simulink model "scd3busMicrogridDroopControlFidelityLevels3Inv"  (R2025b)
settings: Solver=ode15s  StartTime=0.0  StopTime=24  RelTol=1e-3
PreLoadFcn:
  | scd3busMicrogridDroopControlDataFidelityLevels3Inv;
  | 
  | %% Controller variants
  | % Create variant controls for converter controller. Controller has two
  | % different levels of fidelity: Averaged, AveragedPulse, Pulse
  | Averaged = Simulink.VariantExpression;
  | Averaged.Condition = 'fidelity==scd3busMicrogridDroopControl_variants_enum.Low';
  | Pulse = Simulink.VariantExpression;
  | Pulse.Condition = 'fidelity==scd3busMicrogridDroopControl_variants_enum.High';
  | 
  | %% Plant variants
  | % Create variant controls for converter plant. Plant has three different
  | % levels of fidelity.
  | AveragedNonSwitch = Simulink.VariantExpression;
  | AveragedNonSwitch.Condition = 'fidelity==scd3busMicrogridDroopControl_variants_enum.Low';
  | PulseSwitch = Simulink.VariantExpression;
  | PulseSwitch.Condition = 'fidelity==scd3busMicrogridDroopControl_variants_enum.High';
  | 
  | %% Set up variables ready for simulation
  | fidelity = scd3busMicrogridDroopControl_variants_enum.High;
  | Ts = 5e-6;
  | Ts_V = 1e-6;
  | Tsc = 1e-4;
  | Tsc_V = 5e-4;
values from neighbouring files (symbols this model uses):
  consensus_enable = 1    [scd3busMicrogridDroopControlDataFidelityLevels3Inv.m]
  fgrid = 60    [scd3busMicrogridDroopControlDataFidelityLevels.m]    (also in scd3busMicrogridDroopControlDataFidelityLevels3Inv.m)
  Kdroop_fp1 = 0.03/2    (= 0.015)    [scd3busMicrogridDroopControlDataFidelityLevels3Inv.m]
  Kdroop_fp2 = 0.03/2    (= 0.015)    [scd3busMicrogridDroopControlDataFidelityLevels3Inv.m]
  Kdroop_vq1 = 0.05/2    (= 0.025)    [scd3busMicrogridDroopControlDataFidelityLevels3Inv.m]
  Kdroop_vq2 = 0.05/2    (= 0.025)    [scd3busMicrogridDroopControlDataFidelityLevels3Inv.m]
  Ki_vd = 850    [scd3busMicrogridDroopControlDataFidelityLevels.m]    (also in scd3busMicrogridDroopControlDataFidelityLevels3Inv.m)
  Ki_vq = 850    [scd3busMicrogridDroopControlDataFidelityLevels.m]    (also in scd3busMicrogridDroopControlDataFidelityLevels3Inv.m)
  Kp_vd = 0.36    [scd3busMicrogridDroopControlDataFidelityLevels.m]    (also in scd3busMicrogridDroopControlDataFidelityLevels3Inv.m)
  Kp_vq = 0.36    [scd3busMicrogridDroopControlDataFidelityLevels.m]    (also in scd3busMicrogridDroopControlDataFidelityLevels3Inv.m)
  Vdc1 = 1000    [scd3busMicrogridDroopControlDataFidelityLevels.m]    (also in scd3busMicrogridDroopControlDataFidelityLevels3Inv.m)
  Vdc2 = 1000    [scd3busMicrogridDroopControlDataFidelityLevels.m]    (also in scd3busMicrogridDroopControlDataFidelityLevels3Inv.m)
  Vrms = 380    [scd3busMicrogridDroopControlDataFidelityLevels.m]    (also in scd3busMicrogridDroopControlDataFidelityLevels3Inv.m)
undefined symbols (not defined in the file or in its folder): DiscIntNeverNeededParam
libraries: ee_lib x29, nesl_utility x27, fl_lib x15, eeTransforms x4, eeSinusoidalMeasurement x4, slpidlib x4, eePwmGeneratorTwoLevel x2, eePowerMeasurement x2, simulink x2, SignalEditorBlockLib x1
(part 1 of 3)
Description:
  | Three-Phase 3 Bus Low-Inertia Microgrid Droop Control Example
settings Model: SimulationMode=rapid-accelerator  Creator=The MathWorks, Inc.  LastModifiedBy=Alex
settings SolverCC: MaxZcPerStep=1.0
settings DataIOCC: SaveOutput=off  DSMLogging=off  SaveTime=off  ReturnWorkspaceOutputs=off
settings OptimizationCC: ReuseModelBlockBuffer=off
settings DebuggingCC: StateNameClashWarn=warning
settings ModelReferenceCC: EnableRefExpFcnMdlSchedulingChecks=on
settings RTWCC: GPUComputeCapability=3.5
settings SimscapeCC: SimscapeNormalizeSystem=off

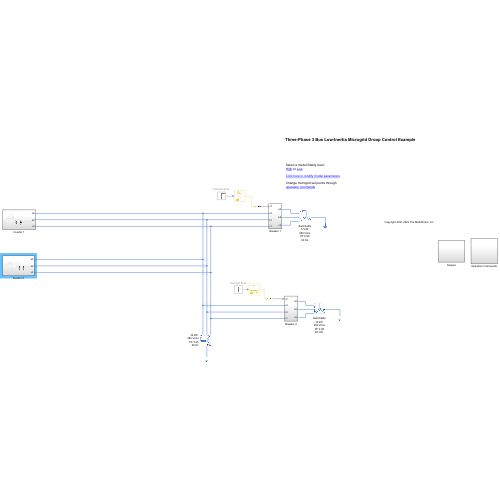
[thumbnail: Simulink's stored preview of the top-level diagram]
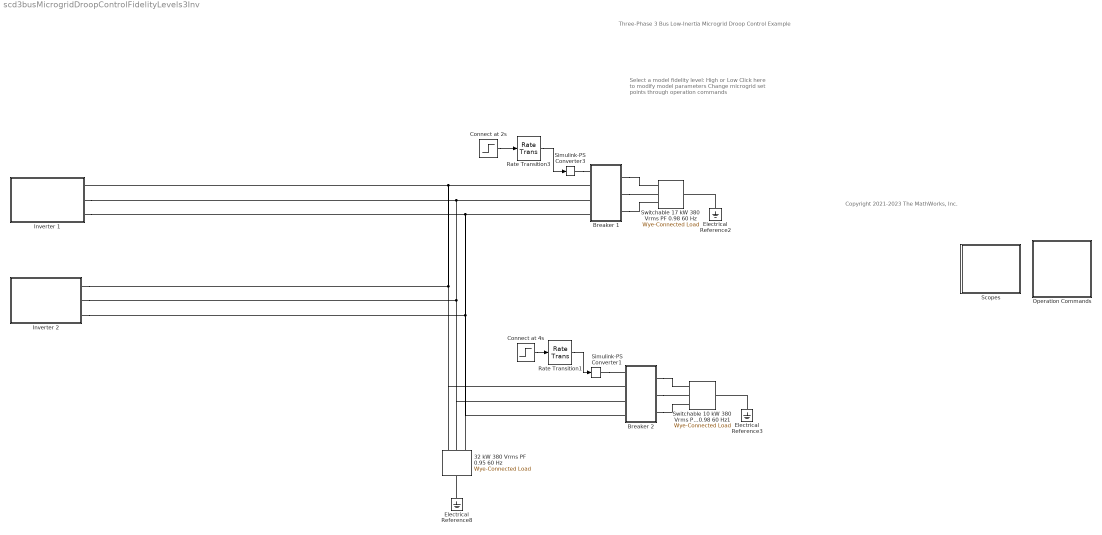
== system scd3busMicrogridDroopControlFidelityLevels3Inv ==
  note: Three-Phase 3 Bus Low-Inertia Microgrid Droop Control Example
  note: Copyright 2021-2023 The MathWorks, Inc.
  note: Select a model fidelity level:
      | High or Low
      |
      | Click here to modify model parameters
      |
      | Change microgrid set points through operation commands
  32 kW 380 Vrms PF 0.95 60 Hz : ee_lib/Passive/RLC Assemblies/Wye-Connected Load  port_option=ee.enum.threePhasePort.expanded  parameterization=2  component_structure=3  component_structure_PQ=ee.enum.rlc.structure.ParallelRL  R=1 Ohm  L=0.001 H  C=1e-6 F  VRated=Vrms V  FRated=fgrid Hz  P=32000 W  Qpos=32000*sqrt(1-0.95^2)/0.95 V*A  Qneg=-3000 V*A  R_parasitic=1e-6 Ohm  G_parasitic=1e-6 1/Ohm  R_parasitic_PQ=1e-6 Ohm  G_parasitic_PQ=1e-6 1/Ohm  Vmag0=380 V  Vang0=0 deg  Freq0=60 Hz  IL_specify=on  IL_priority=High  IL=[ 0 0 0 ] A  IL_nominal_specify=off  IL_nominal_value=1  IL_nominal_unit=A  VC_specify=on  VC_priority=High  VC=[ 0 0 0 ] V  VC_nominal_specify=off  VC_nominal_value=1  VC_nominal_unit=V
      settings: InternalSimscapePortConfiguration="{\"Bottom\":[],\"Left\":[{\"id\":\"a\",\"label\":\"a\",\"type\":\"foundation.electrical.electrical\"},{\"id\":\"b\",\"label\":\"b\",\"type\":\"foundation.electrical.electrical\"},{\"id\":\"c\",\"label\":\"c\",\"type\":\"foundation.electrical.electrical\"}],\"Right\":[{\"id\":\"n\",\"label\":\"n\",\"type\":\"foundation.electrical.electrical\"}],\"Top\":[]}"
  Breaker 1 : Subsystem
  Breaker 2 : Subsystem
  Connect at 2s : Step  Time=6  SampleTime=0
  Connect at 4s : Step  Time=10  SampleTime=0
  Electrical Reference2 : fl_lib/Electrical/Electrical Elements/Electrical Reference
  Electrical Reference3 : fl_lib/Electrical/Electrical Elements/Electrical Reference
  Electrical Reference8 : fl_lib/Electrical/Electrical Elements/Electrical Reference
  Inverter 1 : Subsystem
  Inverter 2 : Subsystem
  Operation Commands : Subsystem
  Rate Transition1 : RateTransition  Integrity=off  OutPortSampleTimeOpt=Inherit
  Rate Transition3 : RateTransition  Integrity=off  OutPortSampleTimeOpt=Inherit
  Scopes : Subsystem
  Simulink-PS Converter1 : nesl_utility/Simulink-PS Converter  PhysicalDomain=network_engine_domain  SubClassName=ps_input  LeftPortType=input  RightPortType=output  PseudoPeriodic=off  Frequencies=[]  NoiseDistribution=none  NoiseParameters=[]  Unit=1  AffineConversion=off  FilteringAndDerivatives=provide  SimscapeFilterOrder=1  InputFilterTimeConstant=0.001  UdotUserProvided=0
  Simulink-PS Converter3 : nesl_utility/Simulink-PS Converter  PhysicalDomain=network_engine_domain  SubClassName=ps_input  LeftPortType=input  RightPortType=output  PseudoPeriodic=off  Frequencies=[]  NoiseDistribution=none  NoiseParameters=[]  Unit=1  AffineConversion=off  FilteringAndDerivatives=provide  SimscapeFilterOrder=1  InputFilterTimeConstant=0.001  UdotUserProvided=0
  Switchable 10 kW 380 Vrms PF 0.98 60 Hz1 : ee_lib/Passive/RLC Assemblies/Wye-Connected Load  port_option=ee.enum.threePhasePort.expanded  parameterization=2  component_structure=3  component_structure_PQ=ee.enum.rlc.structure.ParallelRL  R=1 Ohm  L=0.001 H  C=1e-6 F  VRated=Vrms V  FRated=fgrid Hz  P=10000 W  Qpos=10000*sqrt(1-0.98^2)/0.98 V*A  Qneg=-3000 V*A  R_parasitic=1e-6 Ohm  G_parasitic=1e-6 1/Ohm  R_parasitic_PQ=1e-6 Ohm  G_parasitic_PQ=1e-6 1/Ohm  Vmag0=380 V  Vang0=0 deg  Freq0=60 Hz  IL_specify=on  IL_priority=High  IL=[ 0 0 0 ] A  IL_nominal_specify=off  IL_nominal_value=1  IL_nominal_unit=A  VC_specify=on  VC_priority=High  VC=[ 0 0 0 ] V  VC_nominal_specify=off  VC_nominal_value=1  VC_nominal_unit=V
      settings: InternalSimscapePortConfiguration="{\"Bottom\":[],\"Left\":[{\"id\":\"a\",\"label\":\"a\",\"type\":\"foundation.electrical.electrical\"},{\"id\":\"b\",\"label\":\"b\",\"type\":\"foundation.electrical.electrical\"},{\"id\":\"c\",\"label\":\"c\",\"type\":\"foundation.electrical.electrical\"}],\"Right\":[{\"id\":\"n\",\"label\":\"n\",\"type\":\"foundation.electrical.electrical\"}],\"Top\":[]}"
  Switchable 17 kW 380 Vrms PF 0.98 60 Hz : ee_lib/Passive/RLC Assemblies/Wye-Connected Load  port_option=ee.enum.threePhasePort.expanded  parameterization=2  component_structure=3  component_structure_PQ=ee.enum.rlc.structure.ParallelRL  R=1 Ohm  L=0.001 H  C=1e-6 F  VRated=Vrms V  FRated=fgrid Hz  P=17000 W  Qpos=17000*sqrt(1-0.98^2)/0.98 V*A  Qneg=-3000 V*A  R_parasitic=1e-6 Ohm  G_parasitic=1e-6 1/Ohm  R_parasitic_PQ=1e-6 Ohm  G_parasitic_PQ=1e-6 1/Ohm  Vmag0=380 V  Vang0=0 deg  Freq0=60 Hz  IL_specify=on  IL_priority=High  IL=[ 0 0 0 ] A  IL_nominal_specify=off  IL_nominal_value=1  IL_nominal_unit=A  VC_specify=on  VC_priority=High  VC=[ 0 0 0 ] V  VC_nominal_specify=off  VC_nominal_value=1  VC_nominal_unit=V
      settings: InternalSimscapePortConfiguration="{\"Bottom\":[],\"Left\":[{\"id\":\"a\",\"label\":\"a\",\"type\":\"foundation.electrical.electrical\"},{\"id\":\"b\",\"label\":\"b\",\"type\":\"foundation.electrical.electrical\"},{\"id\":\"c\",\"label\":\"c\",\"type\":\"foundation.electrical.electrical\"}],\"Right\":[{\"id\":\"n\",\"label\":\"n\",\"type\":\"foundation.electrical.electrical\"}],\"Top\":[]}"
  wires:
  Rate Transition3/1 -> Simulink-PS Converter3/1
  Connect at 2s/1 -> Rate Transition3/1
  Connect at 4s/1 -> Rate Transition1/1
  Rate Transition1/1 -> Simulink-PS Converter1/1
  connections:
  Breaker 1/LConn4 -- Inverter 2/RConn3 -- 32 kW 380 Vrms PF 0.95 60 Hz/LConn3 -- Breaker 2/LConn4 -- Inverter 1/RConn3
  Electrical Reference2/LConn1 -- Switchable 17 kW 380 Vrms PF 0.98 60 Hz/RConn1
  Breaker 1/RConn2 -- Switchable 17 kW 380 Vrms PF 0.98 60 Hz/LConn2
  Electrical Reference8/LConn1 -- 32 kW 380 Vrms PF 0.95 60 Hz/RConn1
  Simulink-PS Converter3/RConn1 -- Breaker 1/LConn1
  Breaker 1/RConn3 -- Switchable 17 kW 380 Vrms PF 0.98 60 Hz/LConn3
  Breaker 1/RConn1 -- Switchable 17 kW 380 Vrms PF 0.98 60 Hz/LConn1
  Breaker 2/RConn2 -- Switchable 10 kW 380 Vrms PF 0.98 60 Hz1/LConn2
  Electrical Reference3/LConn1 -- Switchable 10 kW 380 Vrms PF 0.98 60 Hz1/RConn1
  Breaker 2/RConn3 -- Switchable 10 kW 380 Vrms PF 0.98 60 Hz1/LConn3
  Breaker 2/RConn1 -- Switchable 10 kW 380 Vrms PF 0.98 60 Hz1/LConn1
  Simulink-PS Converter1/RConn1 -- Breaker 2/LConn1
  Breaker 1/LConn3 -- Inverter 1/RConn2 -- Breaker 2/LConn3 -- 32 kW 380 Vrms PF 0.95 60 Hz/LConn2 -- Inverter 2/RConn2
  Breaker 1/LConn2 -- Inverter 2/RConn1 -- 32 kW 380 Vrms PF 0.95 60 Hz/LConn1 -- Breaker 2/LConn2 -- Inverter 1/RConn1

== system scd3busMicrogridDroopControlFidelityLevels3Inv/Breaker 1 ==
  SPST Switch : ee_lib/Switches & Breakers/SPST Switch  R_closed=0.01 Ohm  G_open=1e-6 S  Threshold=0.5 V  Width=0 V  model_dynamics=0  t_on=1e-3 s  t_off=1e-3 s  initial_vT=0 V
      settings: InternalSimscapePortConfiguration="{\"Bottom\":[],\"Left\":[{\"id\":\"vT\",\"label\":\"vT\",\"type\":\"input\"},{\"id\":\"p\",\"label\":\"\",\"type\":\"foundation.electrical.electrical\"}],\"Right\":[{\"id\":\"n\",\"label\":\"\",\"type\":\"foundation.electrical.electrical\"}],\"Top\":[]}"
  SPST Switch1 : ee_lib/Switches & Breakers/SPST Switch  R_closed=0.01 Ohm  G_open=1e-6 S  Threshold=0.5 V  Width=0 V  model_dynamics=0  t_on=1e-3 s  t_off=1e-3 s  initial_vT=0 V
      settings: InternalSimscapePortConfiguration="{\"Bottom\":[],\"Left\":[{\"id\":\"vT\",\"label\":\"vT\",\"type\":\"input\"},{\"id\":\"p\",\"label\":\"\",\"type\":\"foundation.electrical.electrical\"}],\"Right\":[{\"id\":\"n\",\"label\":\"\",\"type\":\"foundation.electrical.electrical\"}],\"Top\":[]}"
  SPST Switch2 : ee_lib/Switches & Breakers/SPST Switch  R_closed=0.01 Ohm  G_open=1e-6 S  Threshold=0.5 V  Width=0 V  model_dynamics=0  t_on=1e-3 s  t_off=1e-3 s  initial_vT=0 V
      settings: InternalSimscapePortConfiguration="{\"Bottom\":[],\"Left\":[{\"id\":\"vT\",\"label\":\"vT\",\"type\":\"input\"},{\"id\":\"p\",\"label\":\"\",\"type\":\"foundation.electrical.electrical\"}],\"Right\":[{\"id\":\"n\",\"label\":\"\",\"type\":\"foundation.electrical.electrical\"}],\"Top\":[]}"
  vT : PMIOPort  Side=Left
  a1 : PMIOPort  Port=2  Side=Left
  b1 : PMIOPort  Port=3  Side=Left
  c1 : PMIOPort  Port=4  Side=Left
  a2 : PMIOPort  Port=5  Side=Right
  b2 : PMIOPort  Port=6  Side=Right
  c2 : PMIOPort  Port=7  Side=Right
  connections:
  SPST Switch1/RConn1 -- b2/RConn1
  SPST Switch2/RConn1 -- a2/RConn1
  SPST Switch/LConn1 -- SPST Switch1/LConn1 -- vT/RConn1 -- SPST Switch2/LConn1
  SPST Switch/RConn1 -- c2/RConn1
  SPST Switch2/LConn2 -- a1/RConn1
  SPST Switch/LConn2 -- c1/RConn1
  SPST Switch1/LConn2 -- b1/RConn1

== system scd3busMicrogridDroopControlFidelityLevels3Inv/Breaker 2 ==
  SPST Switch : ee_lib/Switches & Breakers/SPST Switch  R_closed=0.01 Ohm  G_open=1e-6 S  Threshold=0.5 V  Width=0 V  model_dynamics=0  t_on=1e-3 s  t_off=1e-3 s  initial_vT=0 V
      settings: InternalSimscapePortConfiguration="{\"Bottom\":[],\"Left\":[{\"id\":\"vT\",\"label\":\"vT\",\"type\":\"input\"},{\"id\":\"p\",\"label\":\"\",\"type\":\"foundation.electrical.electrical\"}],\"Right\":[{\"id\":\"n\",\"label\":\"\",\"type\":\"foundation.electrical.electrical\"}],\"Top\":[]}"
  SPST Switch1 : ee_lib/Switches & Breakers/SPST Switch  R_closed=0.01 Ohm  G_open=1e-6 S  Threshold=0.5 V  Width=0 V  model_dynamics=0  t_on=1e-3 s  t_off=1e-3 s  initial_vT=0 V
      settings: InternalSimscapePortConfiguration="{\"Bottom\":[],\"Left\":[{\"id\":\"vT\",\"label\":\"vT\",\"type\":\"input\"},{\"id\":\"p\",\"label\":\"\",\"type\":\"foundation.electrical.electrical\"}],\"Right\":[{\"id\":\"n\",\"label\":\"\",\"type\":\"foundation.electrical.electrical\"}],\"Top\":[]}"
  SPST Switch2 : ee_lib/Switches & Breakers/SPST Switch  R_closed=0.01 Ohm  G_open=1e-6 S  Threshold=0.5 V  Width=0 V  model_dynamics=0  t_on=1e-3 s  t_off=1e-3 s  initial_vT=0 V
      settings: InternalSimscapePortConfiguration="{\"Bottom\":[],\"Left\":[{\"id\":\"vT\",\"label\":\"vT\",\"type\":\"input\"},{\"id\":\"p\",\"label\":\"\",\"type\":\"foundation.electrical.electrical\"}],\"Right\":[{\"id\":\"n\",\"label\":\"\",\"type\":\"foundation.electrical.electrical\"}],\"Top\":[]}"
  vT : PMIOPort  Side=Left
  a1 : PMIOPort  Port=2  Side=Left
  b1 : PMIOPort  Port=3  Side=Left
  c1 : PMIOPort  Port=4  Side=Left
  a2 : PMIOPort  Port=5  Side=Right
  b2 : PMIOPort  Port=6  Side=Right
  c2 : PMIOPort  Port=7  Side=Right
  connections:
  SPST Switch1/RConn1 -- b2/RConn1
  SPST Switch2/RConn1 -- a2/RConn1
  SPST Switch/LConn1 -- SPST Switch1/LConn1 -- vT/RConn1 -- SPST Switch2/LConn1
  SPST Switch/RConn1 -- c2/RConn1
  SPST Switch2/LConn2 -- a1/RConn1
  SPST Switch/LConn2 -- c1/RConn1
  SPST Switch1/LConn2 -- b1/RConn1

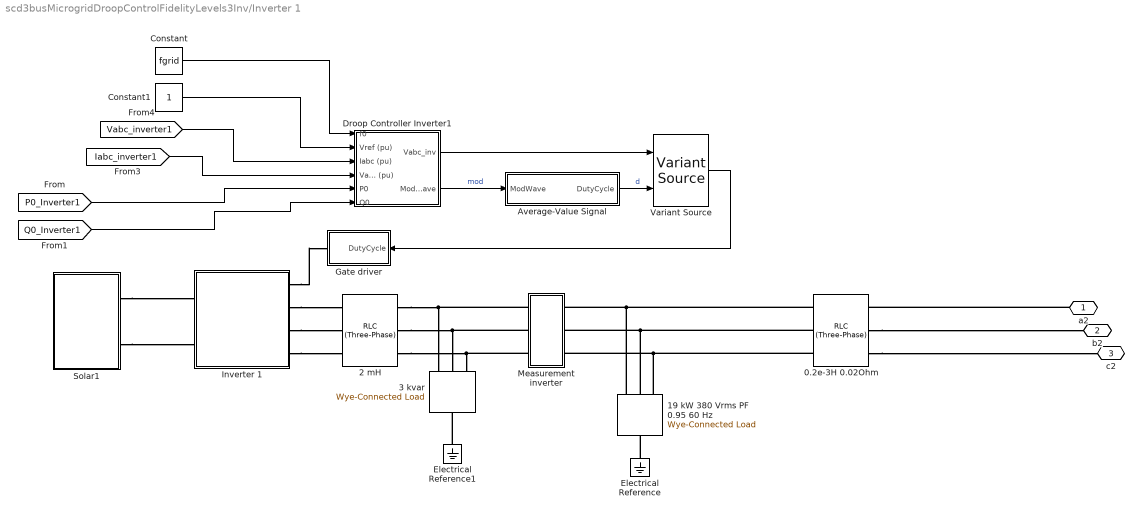
== system scd3busMicrogridDroopControlFidelityLevels3Inv/Inverter 1 ==
  0.2e-3H 0.02Ohm : ee_lib/Passive/RLC Assemblies/RLC (Three-Phase)  port_option=ee.enum.threePhasePort.expanded  component_structure=ee.enum.rlc.structure.SeriesRL  R=0.02 Ohm  L=0.2e-3 H  C=1 F  R_parasitic=1e-6 Ohm  G_parasitic=1e-6 1/Ohm  IL_specify=on  IL_priority=High  IL=[0, 0, 0] A  IL_nominal_specify=off  IL_nominal_value=1  IL_nominal_unit=A  VC_specify=on  VC_priority=High  VC=[0, 0, 0] V  VC_nominal_specify=off  VC_nominal_value=1  VC_nominal_unit=V
      settings: InternalSimscapePortConfiguration="{\"Bottom\":[],\"Left\":[{\"id\":\"a1\",\"label\":\"a1\",\"type\":\"foundation.electrical.electrical\"},{\"id\":\"b1\",\"label\":\"b1\",\"type\":\"foundation.electrical.electrical\"},{\"id\":\"c1\",\"label\":\"c1\",\"type\":\"foundation.electrical.electrical\"}],\"Right\":[{\"id\":\"a2\",\"label\":\"a2\",\"type\":\"foundation.electrical.electrical\"},{\"id\":\"b2\",\"label\":\"b2\",\"type\":\"foundation.electrical.electrical\"},{\"id\":\"c2\",\"label\":\"c2\",\"type\":\"foundation.electrical.electrical\"}],\"Top\":[]}"
  19 kW 380 Vrms PF 0.95 60 Hz : ee_lib/Passive/RLC Assemblies/Wye-Connected Load  port_option=ee.enum.threePhasePort.expanded  parameterization=2  component_structure=3  component_structure_PQ=ee.enum.rlc.structure.ParallelRL  R=1 Ohm  L=0.001 H  C=1e-6 F  VRated=Vrms V  FRated=fgrid Hz  P=19000 W  Qpos=19000*sqrt(1-0.95^2)/0.95 V*A  Qneg=-3000 V*A  R_parasitic=1e-6 Ohm  G_parasitic=1e-6 1/Ohm  R_parasitic_PQ=1e-6 Ohm  G_parasitic_PQ=1e-6 1/Ohm  Vmag0=380 V  Vang0=0 deg  Freq0=60 Hz  IL_specify=on  IL_priority=High  IL=[ 0 0 0 ] A  IL_nominal_specify=off  IL_nominal_value=1  IL_nominal_unit=A  VC_specify=on  VC_priority=High  VC=[ 0 0 0 ] V  VC_nominal_specify=off  VC_nominal_value=1  VC_nominal_unit=V
      settings: InternalSimscapePortConfiguration="{\"Bottom\":[],\"Left\":[{\"id\":\"a\",\"label\":\"a\",\"type\":\"foundation.electrical.electrical\"},{\"id\":\"b\",\"label\":\"b\",\"type\":\"foundation.electrical.electrical\"},{\"id\":\"c\",\"label\":\"c\",\"type\":\"foundation.electrical.electrical\"}],\"Right\":[{\"id\":\"n\",\"label\":\"n\",\"type\":\"foundation.electrical.electrical\"}],\"Top\":[]}"
  "2 mH " : ee_lib/Passive/RLC Assemblies/RLC (Three-Phase)  port_option=ee.enum.threePhasePort.expanded  component_structure=ee.enum.rlc.structure.SeriesRL  R=0.02 Ohm  L=0.002 H  C=1 F  R_parasitic=1e-6 Ohm  G_parasitic=1e-6 1/Ohm  IL_specify=on  IL_priority=High  IL=[0, 0, 0] A  IL_nominal_specify=off  IL_nominal_value=1  IL_nominal_unit=A  VC_specify=on  VC_priority=High  VC=[0, 0, 0] V  VC_nominal_specify=off  VC_nominal_value=1  VC_nominal_unit=V
      settings: InternalSimscapePortConfiguration="{\"Bottom\":[],\"Left\":[{\"id\":\"a1\",\"label\":\"a1\",\"type\":\"foundation.electrical.electrical\"},{\"id\":\"b1\",\"label\":\"b1\",\"type\":\"foundation.electrical.electrical\"},{\"id\":\"c1\",\"label\":\"c1\",\"type\":\"foundation.electrical.electrical\"}],\"Right\":[{\"id\":\"a2\",\"label\":\"a2\",\"type\":\"foundation.electrical.electrical\"},{\"id\":\"b2\",\"label\":\"b2\",\"type\":\"foundation.electrical.electrical\"},{\"id\":\"c2\",\"label\":\"c2\",\"type\":\"foundation.electrical.electrical\"}],\"Top\":[]}"
  3 kvar : ee_lib/Passive/RLC Assemblies/Wye-Connected Load  port_option=ee.enum.threePhasePort.expanded  parameterization=2  component_structure=3  component_structure_PQ=3  R=1 Ohm  L=0.001 H  C=1e-6 F  VRated=Vrms V  FRated=fgrid Hz  P=0 W  Qpos=0 V*A  Qneg=-3000 V*A  R_parasitic=1e-6 Ohm  G_parasitic=1e-6 1/Ohm  R_parasitic_PQ=1e-6 Ohm  G_parasitic_PQ=1e-6 1/Ohm  Vmag0=380 V  Vang0=0 deg  Freq0=60 Hz  IL_specify=on  IL_priority=High  IL=[ 0 0 0 ] A  IL_nominal_specify=off  IL_nominal_value=1  IL_nominal_unit=A  VC_specify=on  VC_priority=High  VC=[ 0 0 0 ] V  VC_nominal_specify=off  VC_nominal_value=1  VC_nominal_unit=V
      settings: InternalSimscapePortConfiguration="{\"Bottom\":[],\"Left\":[{\"id\":\"a\",\"label\":\"a\",\"type\":\"foundation.electrical.electrical\"},{\"id\":\"b\",\"label\":\"b\",\"type\":\"foundation.electrical.electrical\"},{\"id\":\"c\",\"label\":\"c\",\"type\":\"foundation.electrical.electrical\"}],\"Right\":[{\"id\":\"n\",\"label\":\"n\",\"type\":\"foundation.electrical.electrical\"}],\"Top\":[]}"
  Average-Value Signal : Subsystem
  Constant : Constant  Value=fgrid
  Constant1 : Constant
  Droop Controller Inverter1 : Subsystem
  Electrical Reference : fl_lib/Electrical/Electrical Elements/Electrical Reference
  Electrical Reference1 : fl_lib/Electrical/Electrical Elements/Electrical Reference
  Gate driver : Subsystem
  Inverter 1 : Subsystem  Variant=on  VariantControl=Choice
  Measurement inverter : Subsystem
  Solar1 : Subsystem
  Variant Source : VariantSource  ShowConditionOnBlock=on  VariantControls={Pulse, Averaged}
  a2 : PMIOPort  Side=Right
  b2 : PMIOPort  Port=2  Side=Right
  c2 : PMIOPort  Port=3  Side=Right
  wires:
  Average-Value Signal/1(DutyCycle) -> Variant Source/2  "d"
  Droop Controller Inverter1/2(ModWave) -> Average-Value Signal/1(ModWave)  "mod"
  [Vabc_inverter1] -> Droop Controller Inverter1/3(Iabc (pu))
  Constant/1 -> Droop Controller Inverter1/1(f0)
  [Iabc_inverter1] -> Droop Controller Inverter1/4(Vabc (pu))
  Variant Source/1 -> Gate driver/1(DutyCycle)
  Droop Controller Inverter1/1(Vabc_inv) -> Variant Source/1
  Constant1/1 -> Droop Controller Inverter1/2(Vref (pu))
  [Q0_Inverter1] -> Droop Controller Inverter1/6(Q0)
  [P0_Inverter1] -> Droop Controller Inverter1/5(P0)
  connections:
  Measurement inverter/LConn1 -- "2 mH "/RConn1 -- 3 kvar/LConn1
  19 kW 380 Vrms PF 0.95 60 Hz/LConn1 -- 0.2e-3H 0.02Ohm/LConn1 -- Measurement inverter/RConn1
  19 kW 380 Vrms PF 0.95 60 Hz/LConn3 -- 0.2e-3H 0.02Ohm/LConn3 -- Measurement inverter/RConn3
  Inverter 1/LConn2 -- "2 mH "/LConn1
  Electrical Reference1/LConn1 -- 3 kvar/RConn1
  0.2e-3H 0.02Ohm/RConn3 -- c2/RConn1
  Solar1/RConn2 -- Inverter 1/RConn2
  Measurement inverter/LConn2 -- "2 mH "/RConn2 -- 3 kvar/LConn2
  Solar1/RConn1 -- Inverter 1/RConn1
  Inverter 1/LConn4 -- "2 mH "/LConn3
  19 kW 380 Vrms PF 0.95 60 Hz/LConn2 -- 0.2e-3H 0.02Ohm/LConn2 -- Measurement inverter/RConn2
  Inverter 1/LConn3 -- "2 mH "/LConn2
  Electrical Reference/LConn1 -- 19 kW 380 Vrms PF 0.95 60 Hz/RConn1
  Measurement inverter/LConn3 -- "2 mH "/RConn3 -- 3 kvar/LConn3
  Inverter 1/LConn1 -- Gate driver/RConn1
  a2/RConn1 -- 0.2e-3H 0.02Ohm/RConn1
  0.2e-3H 0.02Ohm/RConn2 -- b2/RConn1

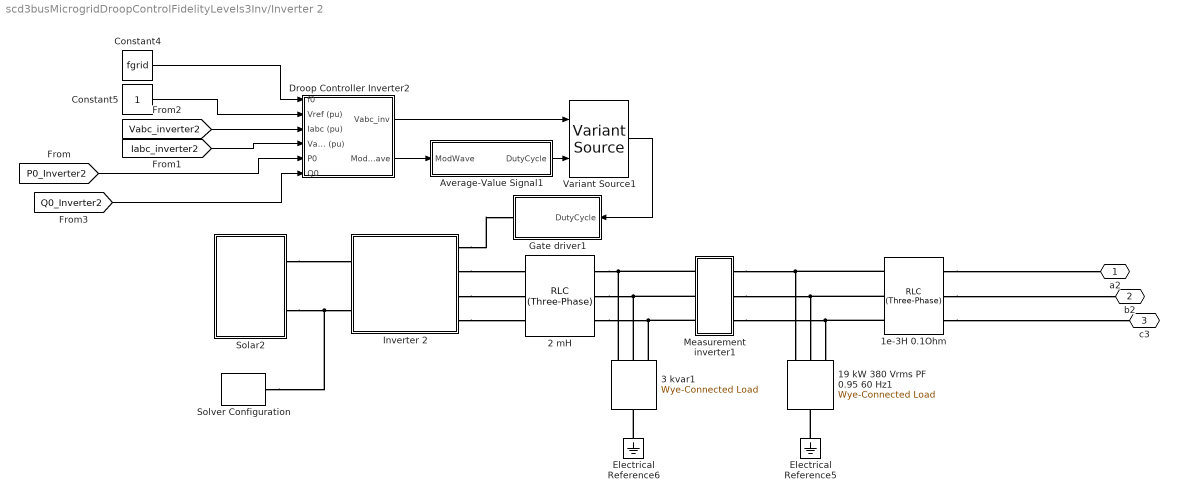
== system scd3busMicrogridDroopControlFidelityLevels3Inv/Inverter 2 ==
  19 kW 380 Vrms PF 0.95 60 Hz1 : ee_lib/Passive/RLC Assemblies/Wye-Connected Load  port_option=ee.enum.threePhasePort.expanded  parameterization=2  component_structure=1  component_structure_PQ=ee.enum.rlc.structure.ParallelRL  R=1 Ohm  L=0.001 H  C=1e-6 F  VRated=Vrms V  FRated=fgrid Hz  P=19000 W  Qpos=19000*sqrt(1-0.95^2)/0.95 V*A  Qneg=-3000 V*A  R_parasitic=1e-6 Ohm  G_parasitic=1e-6 1/Ohm  R_parasitic_PQ=1e-6 Ohm  G_parasitic_PQ=1e-6 1/Ohm  Vmag0=380 V  Vang0=0 deg  Freq0=60 Hz  IL_specify=on  IL_priority=High  IL=[ 0 0 0 ] A  IL_nominal_specify=off  IL_nominal_value=1  IL_nominal_unit=A  VC_specify=on  VC_priority=High  VC=[ 0 0 0 ] V  VC_nominal_specify=off  VC_nominal_value=1  VC_nominal_unit=V
      settings: InternalSimscapePortConfiguration="{\"Bottom\":[],\"Left\":[{\"id\":\"a\",\"label\":\"a\",\"type\":\"foundation.electrical.electrical\"},{\"id\":\"b\",\"label\":\"b\",\"type\":\"foundation.electrical.electrical\"},{\"id\":\"c\",\"label\":\"c\",\"type\":\"foundation.electrical.electrical\"}],\"Right\":[{\"id\":\"n\",\"label\":\"n\",\"type\":\"foundation.electrical.electrical\"}],\"Top\":[]}"
  1e-3H 0.1Ohm : ee_lib/Passive/RLC Assemblies/RLC (Three-Phase)  port_option=ee.enum.threePhasePort.expanded  component_structure=ee.enum.rlc.structure.SeriesRL  R=0.1 Ohm  L=1e-3 H  C=1 F  R_parasitic=1e-6 Ohm  G_parasitic=1e-6 1/Ohm  IL_specify=on  IL_priority=High  IL=[0, 0, 0] A  IL_nominal_specify=off  IL_nominal_value=1  IL_nominal_unit=A  VC_specify=on  VC_priority=High  VC=[0, 0, 0] V  VC_nominal_specify=off  VC_nominal_value=1  VC_nominal_unit=V
      settings: InternalSimscapePortConfiguration="{\"Bottom\":[],\"Left\":[{\"id\":\"a1\",\"label\":\"a1\",\"type\":\"foundation.electrical.electrical\"},{\"id\":\"b1\",\"label\":\"b1\",\"type\":\"foundation.electrical.electrical\"},{\"id\":\"c1\",\"label\":\"c1\",\"type\":\"foundation.electrical.electrical\"}],\"Right\":[{\"id\":\"a2\",\"label\":\"a2\",\"type\":\"foundation.electrical.electrical\"},{\"id\":\"b2\",\"label\":\"b2\",\"type\":\"foundation.electrical.electrical\"},{\"id\":\"c2\",\"label\":\"c2\",\"type\":\"foundation.electrical.electrical\"}],\"Top\":[]}"
  2 mH : ee_lib/Passive/RLC Assemblies/RLC (Three-Phase)  port_option=ee.enum.threePhasePort.expanded  component_structure=ee.enum.rlc.structure.SeriesRL  R=0.02 Ohm  L=0.002 H  C=1 F  R_parasitic=1e-6 Ohm  G_parasitic=1e-6 1/Ohm  IL_specify=on  IL_priority=High  IL=[0, 0, 0] A  IL_nominal_specify=off  IL_nominal_value=1  IL_nominal_unit=A  VC_specify=on  VC_priority=High  VC=[0, 0, 0] V  VC_nominal_specify=off  VC_nominal_value=1  VC_nominal_unit=V
      settings: InternalSimscapePortConfiguration="{\"Bottom\":[],\"Left\":[{\"id\":\"a1\",\"label\":\"a1\",\"type\":\"foundation.electrical.electrical\"},{\"id\":\"b1\",\"label\":\"b1\",\"type\":\"foundation.electrical.electrical\"},{\"id\":\"c1\",\"label\":\"c1\",\"type\":\"foundation.electrical.electrical\"}],\"Right\":[{\"id\":\"a2\",\"label\":\"a2\",\"type\":\"foundation.electrical.electrical\"},{\"id\":\"b2\",\"label\":\"b2\",\"type\":\"foundation.electrical.electrical\"},{\"id\":\"c2\",\"label\":\"c2\",\"type\":\"foundation.electrical.electrical\"}],\"Top\":[]}"
  3 kvar1 : ee_lib/Passive/RLC Assemblies/Wye-Connected Load  port_option=ee.enum.threePhasePort.expanded  parameterization=ee.enum.rlc.parameterization.ratedpower  component_structure=ee.enum.rlc.structure.C  component_structure_PQ=ee.enum.rlc.structure.C  R=1 Ohm  L=0.001 H  C=1e-6 F  VRated=Vrms V  FRated=fgrid Hz  P=0 W  Qpos=0 A*V  Qneg=-3000 A*V  R_parasitic=1e-6 Ohm  G_parasitic=1e-6 1/Ohm  R_parasitic_PQ=1e-6 Ohm  G_parasitic_PQ=1e-6 1/Ohm  Vmag0=380 V  Vang0=0 deg  Freq0=60 Hz  IL_specify=on  IL_priority=High  IL=[ 0 0 0 ] A  IL_nominal_specify=off  IL_nominal_value=1  IL_nominal_unit=A  VC_specify=on  VC_priority=High  VC=[ 0 0 0 ] V  VC_nominal_specify=off  VC_nominal_value=1  VC_nominal_unit=V
      settings: InternalSimscapePortConfiguration="{\"Bottom\":[],\"Left\":[{\"id\":\"a\",\"label\":\"a\",\"type\":\"foundation.electrical.electrical\"},{\"id\":\"b\",\"label\":\"b\",\"type\":\"foundation.electrical.electrical\"},{\"id\":\"c\",\"label\":\"c\",\"type\":\"foundation.electrical.electrical\"}],\"Right\":[{\"id\":\"n\",\"label\":\"n\",\"type\":\"foundation.electrical.electrical\"}],\"Top\":[]}"
  Average-Value Signal1 : Subsystem
  Constant4 : Constant  Value=fgrid
  Constant5 : Constant
  Droop Controller Inverter2 : Subsystem
  Electrical Reference5 : fl_lib/Electrical/Electrical Elements/Electrical Reference
  Electrical Reference6 : fl_lib/Electrical/Electrical Elements/Electrical Reference
  Gate driver1 : Subsystem
  Inverter 2 : Subsystem  Variant=on  VariantControl=Choice
  Measurement inverter1 : Subsystem
  Solar2 : Subsystem
  Solver Configuration : nesl_utility/Solver Configuration  PhysicalDomain=network_engine_domain  SubClassName=solver  LeftPortType=input  RightPortType=generic  Tones=[]  Harmonics=[]  SimulateNoise=off  Profile=off  UseLocalSampling=off  EnableSwitchedLinearOptims=on  FrequencyDomain=off  UseCCode=off  RelTol=0.001  AbsTol=1e-06  MinStep=1e-09  ToWorkspace=off  RevertToSquareIcSolve=off  NumHomotopyIterations=100  PhasorMode=off  PhasorModeNumHarmonics=1  ConsistencySolver=NEWTON_FTOL  IndexReductionMethod=DerivativeReplacement  DoDC=off  ResidualTolerance=1e-09  ConsistencyTolSource=GLOBAL  ConsistencyAbsTol=0.001  ConsistencyRelTol=0.001  ConsistencyTolFactor=0.001  UseLocalSolver=on  LocalSolverChoice=NE_BACKWARD_EULER_ADVANCER  ResolveIndetEquations=on  FunctionEvalNumThread=1  LocalSolverSampleTime=Ts  DoFixedCost=off  MaxNonlinIter=3  MaxModeIter=2  ComputeImpulses=off  ImpulseIterations=1  LinearAlgebra=auto  LinearAlgebraNumThread=0  EquationFormulation=NE_TIME_EF  DelaysMemoryBudget=1024  AutomaticFiltering=on  FilteringTimeConstant=0.001  PartitionStorageMethod=AS_NEEDED  PartitionMemoryBudget=1024  PartitionMethod=FAST  MultibodyUseLocalSolver=off  MultibodyLocalSolverChoice=ODE1  MultibodyLocalSolverSampleTime=0.001
  Variant Source1 : VariantSource  ShowConditionOnBlock=on  VariantControls={Pulse, Averaged}
  a2 : PMIOPort  Side=Right
  b2 : PMIOPort  Port=2  Side=Right
  c3 : PMIOPort  Port=3  Side=Right
  wires:
  Average-Value Signal1/1(DutyCycle) -> Variant Source1/2
  [Iabc_inverter2] -> Droop Controller Inverter2/4(Vabc (pu))
  Variant Source1/1 -> Gate driver1/1(DutyCycle)
  Constant5/1 -> Droop Controller Inverter2/2(Vref (pu))
  Droop Controller Inverter2/1(Vabc_inv) -> Variant Source1/1
  Droop Controller Inverter2/2(ModWave) -> Average-Value Signal1/1(ModWave)
  Constant4/1 -> Droop Controller Inverter2/1(f0)
  [Vabc_inverter2] -> Droop Controller Inverter2/3(Iabc (pu))
  [P0_Inverter2] -> Droop Controller Inverter2/5(P0)
  [Q0_Inverter2] -> Droop Controller Inverter2/6(Q0)
  connections:
  2 mH/RConn2 -- Measurement inverter1/LConn2 -- 3 kvar1/LConn2
  Measurement inverter1/RConn1 -- 1e-3H 0.1Ohm/LConn1 -- 19 kW 380 Vrms PF 0.95 60 Hz1/LConn1
  Measurement inverter1/RConn2 -- 1e-3H 0.1Ohm/LConn2 -- 19 kW 380 Vrms PF 0.95 60 Hz1/LConn2
  1e-3H 0.1Ohm/RConn3 -- c3/RConn1
  2 mH/RConn1 -- Measurement inverter1/LConn1 -- 3 kvar1/LConn1
  Inverter 2/LConn4 -- 2 mH/LConn3
  2 mH/RConn3 -- Measurement inverter1/LConn3 -- 3 kvar1/LConn3
  1e-3H 0.1Ohm/RConn2 -- b2/RConn1
  1e-3H 0.1Ohm/RConn1 -- a2/RConn1
  1e-3H 0.1Ohm/LConn3 -- Measurement inverter1/RConn3 -- 19 kW 380 Vrms PF 0.95 60 Hz1/LConn3
  Inverter 2/LConn3 -- 2 mH/LConn2
  Inverter 2/LConn2 -- 2 mH/LConn1
  Electrical Reference5/LConn1 -- 19 kW 380 Vrms PF 0.95 60 Hz1/RConn1
  Solar2/RConn1 -- Inverter 2/RConn1
  Solar2/RConn2 -- Solver Configuration/RConn1 -- Inverter 2/RConn2
  Inverter 2/LConn1 -- Gate driver1/RConn1
  Electrical Reference6/LConn1 -- 3 kvar1/RConn1

== system scd3busMicrogridDroopControlFidelityLevels3Inv/Operation Commands ==
  Microgrid Operation Scheduler : SignalEditorBlockLib/Signal Editor  FileName=scd3busMicrogridDroopControlSetPoints.mat  ActiveScenario=Scenario  ActiveSignal=P_inverter2  IsBus=off  OutputBusObjectStr=Bus: BusObject  SampleTime=0  Interpolate=off  ZeroCross=off  OutputAfterFinalValue=Setting to zero  Unit=inherit  PreserveSignalName=on  ApplySigPropsToAllScenarios=on  ApplySigPropsToAllSignals=off  SignalPropertySource=Dialog parameters
  tag scope: P0_Inverter1=global, P0_Inverter2=global, P0_Inverter3=global, Q0_Inverter1=global, Q0_Inverter2=global, Q0_Inverter3=global
  wires:
  Microgrid Operation Scheduler/4 -> [Q0_Inverter2]
  Microgrid Operation Scheduler/1 -> [P0_Inverter1]
  Microgrid Operation Scheduler/3 -> [P0_Inverter2]
  Microgrid Operation Scheduler/2 -> [Q0_Inverter1]
  Microgrid Operation Scheduler/5 -> [P0_Inverter3]
  Microgrid Operation Scheduler/6 -> [Q0_Inverter3]

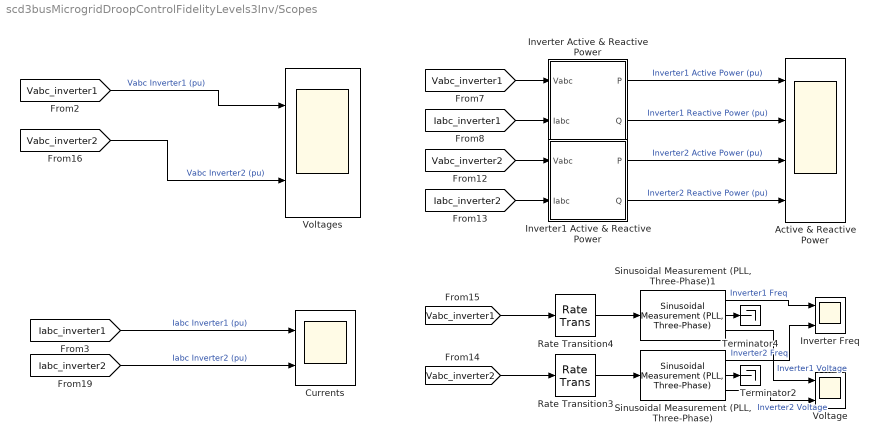
== system scd3busMicrogridDroopControlFidelityLevels3Inv/Scopes ==
  Active & Reactive Power : Scope  NumInputPorts=4
      settings: ActiveDisplayYMinimum=-1.299645784909139  ActiveDisplayYMaximum=1.4039149273407447  DataLoggingDecimation=10
  Currents : Scope  NumInputPorts=2
      settings: ActiveDisplayYMinimum=-5.6609298976060849  ActiveDisplayYMaximum=4.96308312446277  DataLoggingVariableName=ScopeData2
  "Inverter Active & Reactive Power " : Subsystem
  Inverter Freq : Scope  NumInputPorts=2
      settings: ActiveDisplayYMinimum=56.849571603284438  ActiveDisplayYMaximum=67.17364545741404  DataLoggingVariableName=ScopeData2
  Inverter1 Active & Reactive Power : Subsystem
  Rate Transition3 : RateTransition  OutPortSampleTime=Tsc
  Rate Transition4 : RateTransition  OutPortSampleTime=Tsc
  "Sinusoidal Measurement (PLL, Three-Phase)" : eeSinusoidalMeasurement/Sinusoidal Measurement (PLL, Three-Phase)  Kp_LF=150  Ki_LF=150  F0=fgrid  Theta0=0  Ts=Tsc
  "Sinusoidal Measurement (PLL, Three-Phase)1" : eeSinusoidalMeasurement/Sinusoidal Measurement (PLL, Three-Phase)  Kp_LF=150  Ki_LF=150  F0=fgrid  Theta0=0  Ts=Tsc
  Terminator2 : Terminator
  Terminator4 : Terminator
  Voltage : Scope  NumInputPorts=2
      settings: ActiveDisplayYMinimum=0.96870445331736421  ActiveDisplayYMaximum=1.1699365978202856
  Voltages : Scope  NumInputPorts=2
      settings: ActiveDisplayYMinimum=-1.5360989139716028  ActiveDisplayYMaximum=1.53441595827697  DataLoggingVariableName=ScopeData6
  wires:
  [Iabc_inverter1] -> Currents/1  "Iabc Inverter1 (pu)"
  [Vabc_inverter1] -> Voltages/1  "Vabc Inverter1 (pu)"
  [Vabc_inverter1] -> "Inverter Active & Reactive Power "/1(Vabc)
  [Iabc_inverter1] -> "Inverter Active & Reactive Power "/2(Iabc)
  "Inverter Active & Reactive Power "/1(P) -> Active & Reactive Power/1  "Inverter1 Active Power (pu)"
  "Inverter Active & Reactive Power "/2(Q) -> Active & Reactive Power/2  "Inverter1 Reactive Power (pu)"
  Inverter1 Active & Reactive Power/2(Q) -> Active & Reactive Power/4  "Inverter2 Reactive Power (pu)"
  Inverter1 Active & Reactive Power/1(P) -> Active & Reactive Power/3  "Inverter2 Active Power (pu)"
  [Iabc_inverter2] -> Inverter1 Active & Reactive Power/2(Iabc)
  [Vabc_inverter2] -> Inverter1 Active & Reactive Power/1(Vabc)
  Rate Transition3/1 -> "Sinusoidal Measurement (PLL, Three-Phase)"/1
  "Sinusoidal Measurement (PLL, Three-Phase)"/1 -> Inverter Freq/2  "Inverter2 Freq"
  Rate Transition4/1 -> "Sinusoidal Measurement (PLL, Three-Phase)1"/1
  "Sinusoidal Measurement (PLL, Three-Phase)1"/2 -> Terminator4/1
  "Sinusoidal Measurement (PLL, Three-Phase)1"/1 -> Inverter Freq/1  "Inverter1 Freq"
  [Vabc_inverter1] -> Rate Transition4/1
  "Sinusoidal Measurement (PLL, Three-Phase)"/2 -> Terminator2/1
  [Vabc_inverter2] -> Rate Transition3/1
  "Sinusoidal Measurement (PLL, Three-Phase)"/3 -> Voltage/2  "Inverter2 Voltage"
  "Sinusoidal Measurement (PLL, Three-Phase)1"/3 -> Voltage/1  "Inverter1 Voltage"
  [Iabc_inverter2] -> Currents/2  "Iabc Inverter2 (pu)"
  [Vabc_inverter2] -> Voltages/2  "Vabc Inverter2 (pu)"

== system scd3busMicrogridDroopControlFidelityLevels3Inv/Inverter 1/Average-Value Signal ==
  ModWave : Inport
  Bias : Bias  Bias=1  SaturateOnIntegerOverflow=off
  Bias1 : Bias  Bias=1  SaturateOnIntegerOverflow=off
  Gain : Gain  Gain=-1
  Mod. Index1 : Gain  Gain=0.5
  Mux : Mux  Inputs=2
  Rate Transition : RateTransition  OutPortSampleTime=Ts_V
  Selector4 : Selector  InputPortWidth=6  IndexOptions=Index vector (dialog)  Indices=[1 4 2 5 3 6]  OutputSizes=1
  DutyCycle : Outport
  wires:
  Mux/1 -> Selector4/1
  Bias1/1 -> Mux/2
  Selector4/1 -> DutyCycle/1
  Rate Transition/1 -> Bias/1
  Bias/1 -> Mod. Index1/1
  Mod. Index1/1 -> Mux/1, Gain/1
  Gain/1 -> Bias1/1
  ModWave/1 -> Rate Transition/1

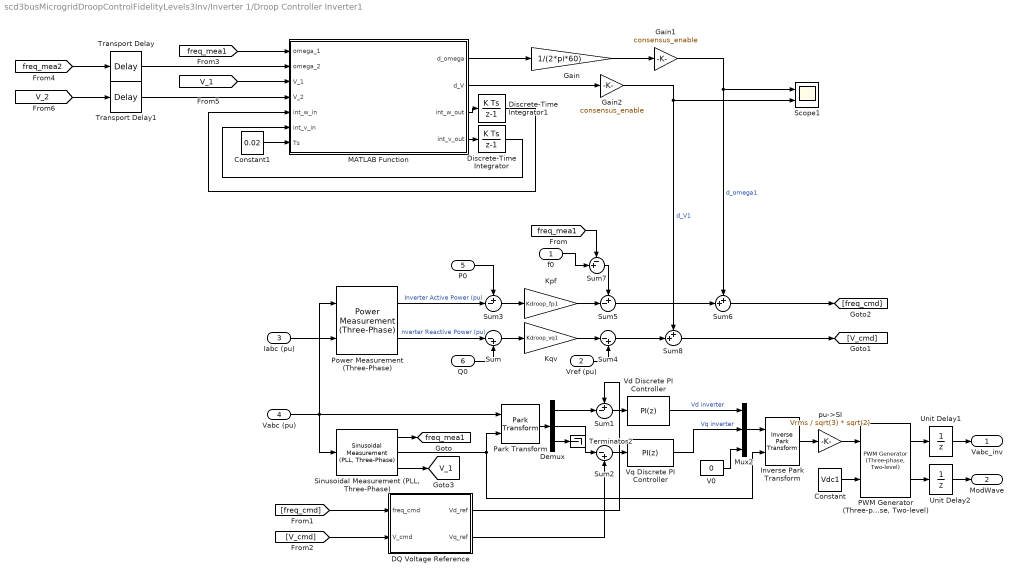
== system scd3busMicrogridDroopControlFidelityLevels3Inv/Inverter 1/Droop Controller Inverter1 ==
  f0 : Inport
  Vref (pu) : Inport  Port=2
  Iabc (pu) : Inport  Port=3
  Vabc (pu) : Inport  Port=4
  P0 : Inport  Port=5
  Q0 : Inport  Port=6
  Constant : Constant  Value=Vdc1
  Constant1 : Constant  Value=0.02
  DQ Voltage Reference : Subsystem
  Demux : Demux  Outputs=3
  Discrete-Time Integrator : DiscreteIntegrator  SampleTime=0.02  ICPrevOutput=DiscIntNeverNeededParam  ICPrevScaledInput=DiscIntNeverNeededParam
  Discrete-Time Integrator1 : DiscreteIntegrator  SampleTime=0.02  ICPrevOutput=DiscIntNeverNeededParam  ICPrevScaledInput=DiscIntNeverNeededParam
  Gain : Gain  Gain=1/(2*pi*60)
  Gain1 : Gain  Gain=consensus_enable
  Gain2 : Gain  Gain=consensus_enable
  Inverse Park Transform : eeTransforms/Inverse Park Transform  AxisAlignment=Q-axis  PowerInvariant=off
  Kpf : Gain  Gain=Kdroop_fp1
  Kqv : Gain  Gain=Kdroop_vq1
  MATLAB Function : MATLAB Function  TreatAsAtomicUnit=on
  Mux2 : Mux  Inputs=3
  "PWM Generator (Three-phase, Two-level)" : eePwmGeneratorTwoLevel/PWM Generator (Three-phase, Two-level)  PWMMode=Continuous PWM (CPWM)  CPWMMode=SPWM: sinusoidal PWM  DPWMMode=60 DPWM: 60 degree discontinuous PWM  fsw=fsw_V  Ts=Ts_V
  Park Transform : eeTransforms/Park Transform  AxisAlignment=Q-axis  PowerInvariant=off
  Power Measurement (Three-Phase) : eePowerMeasurement/Power Measurement (Three-Phase)  LabelModeActiveChoice=Discrete  F=fgrid  K=1  Seq=Positive  Ts=Ts
  Scope1 : Scope  NumInputPorts=2
      settings: ActiveDisplayYMinimum=-0.013262911924324612  ActiveDisplayYMaximum=0.013262911924324612  DataLoggingVariableName=ScopeData3
  "Sinusoidal Measurement (PLL, Three-Phase)" : eeSinusoidalMeasurement/Sinusoidal Measurement (PLL, Three-Phase)  Kp_LF=180  Ki_LF=3200  F0=fgrid  Theta0=0  Ts=Ts_V
  Sum : Sum  Inputs=|-+
  Sum1 : Sum  Inputs=+-|  InputSameDT=on  SaturateOnIntegerOverflow=on  OutDataTypeStr=Inherit: Same as first input
  Sum2 : Sum  Inputs=|-+  InputSameDT=on  SaturateOnIntegerOverflow=on  OutDataTypeStr=Inherit: Same as first input
  Sum3 : Sum  Inputs=+-|
  Sum4 : Sum  Inputs=|-+
  Sum5 : Sum  Inputs=+-|
  Sum6 : Sum  Inputs=++|
  Sum7 : Sum  Inputs=-+|
  Sum8 : Sum  Inputs=++|
  Terminator2 : Terminator
  Transport Delay : TransportDelay  DelayTime=0.1
  Transport Delay1 : TransportDelay  DelayTime=0.1
  Unit Delay1 : UnitDelay  SampleTime=Ts_V  HasFrameUpgradeWarning=on
  Unit Delay2 : UnitDelay  SampleTime=Ts_V  HasFrameUpgradeWarning=on
  V0 : Constant  Value=0
  Vd Discrete PI Controller : slpidlib/PID Controller  Controller=PI  Form=Parallel  TimeDomain=Discrete-time  UseExternalTs=off  SampleTime=Ts_V  IntegratorMethod=Forward Euler  FilterMethod=Forward Euler  ControllerParametersSource=internal  P=Kp_vd  I=Ki_vd  UseKiTs=off  D=0  UseExternalDerivativeSource=off  N=100  UseFilter=on  TunerSelectOption=Transfer Function Based (PID Tuner App)  InitialConditionSource=internal  InitialConditionForIntegrator=0.62  InitialConditionForFilter=0  DifferentiatorICPrevScaledInput=0  ExternalReset=none  TrackingMode=off  Kt=1  LimitOutput=on  SatLimitsSource=internal  UpperSaturationLimit=1  LowerSaturationLimit=0  LinearizeAsGain=on  AntiWindupMode=none  Kb=1  LimitIntegrator=off  UpperIntegratorSaturationLimit=inf  LowerIntegratorSaturationLimit=-inf  POutMin=[]  POutMax=[]  IOutMin=[]  IOutMax=[]  DOutMin=[]  DOutMax=[]  NOutMin=[]  NOutMax=[]  SumOutMin=[]  SumOutMax=[]  SaturationOutMin=[]  SaturationOutMax=[]  PParamMin=[]  PParamMax=[]  IParamMin=[]  IParamMax=[]  DParamMin=[]  DParamMax=[]  NParamMin=[]  NParamMax=[]  KbParamMin=[]  KbParamMax=[]  KtParamMin=[]  KtParamMax=[]  KbOutMin=[]  KbOutMax=[]  KtOutMin=[]  KtOutMax=[]  IntegratorOutMin=[]  IntegratorOutMax=[]  FilterOutMin=[]  FilterOutMax=[]  SumI1OutMin=[]  SumI1OutMax=[]  SumI2OutMin=[]  SumI2OutMax=[]  SumI3OutMin=[]  SumI3OutMax=[]  SumI4OutMin=[]  SumI4OutMax=[]  SumDOutMin=[]  SumDOutMax=[]  DifferentiatorOutMin=[]  DifferentiatorOutMax=[]  FilterDiffOutCoefMin=[]  FilterDiffOutCoefMax=[]  ReciprocalOutMin=[]  ReciprocalOutMax=[]  SumDenOutMin=[]  SumDenOutMax=[]  SumNumOutMin=[]  SumNumOutMax=[]  DivideOutMin=[]  DivideOutMax=[]  UdiffTsProdOutMin=[]  UdiffTsProdOutMax=[]  NTsProdOutMin=[]  NTsProdOutMax=[]  UintegralTsProdOutMin=[]  UintegralTsProdOutMax=[]  UngainTsProdOutMin=[]  UngainTsProdOutMax=[]  ClampingZeroOutDataTypeStr=Inherit: Inherit via back propagation  ClampingZeroOutMin=[]  ClampingZeroOutMax=[]  FilterDenConstantOutDataTypeStr=Inherit: Inherit via back propagation  FilterDenConstantOutMin=[]  FilterDenConstantOutMax=[]  PCopyOutDataTypeStr=Inherit: Inherit via back propagation  PCopyOutMin=[]  PCopyOutMax=[]  NCopyOutDataTypeStr=Inherit: Inherit via back propagation  NCopyOutMin=[]  NCopyOutMax=[]  IntegratorContinuousStateAttributes=''  IntegratorStateMustResolveToSignalObject=off  IntegratorRTWStateStorageClass=Auto  FilterContinuousStateAttributes=''  FilterStateMustResolveToSignalObject=off  FilterRTWStateStorageClass=Auto  ParallelPVariant=InternalParameters  IdealPVariant=Disabled  IVariant=InternalParameters  DVariant=Disabled  IntegratorVariant=Discrete  SatVariant=Enabled  AWVariant=Passthrough  PCopyVariant=Disabled  TRVariant=Disabled  FdbkBlocksVariant=Forward  IdealPFdbkVariant=Disabled  SatFdbkVariant=Disabled  DerivativeFilterVariant=Disabled  NVariant=Disabled  NCopyVariant=Disabled_SignalSpec  FilterICVariant=Disabled  IntegratorICVariant=InternalICs  ExternalResetVariant=Disabled  TRSumVariant=Passthrough  SumFdbkVariant=Disabled  SumVariant=Sum_PI  TsampFilterVariant=InternalTs  TsampNgainVariant=Passthrough  TsampIntegralVariant=Disabled_SignalSpec  ExternalSaturationOutDataTypeStr=Inherit: Same as second input  DerivativeSourceVariant=Disabled  PreIntVariant=InternalPreInt
  Vq Discrete PI Controller : slpidlib/PID Controller  Controller=PI  Form=Parallel  TimeDomain=Discrete-time  UseExternalTs=off  SampleTime=Ts_V  IntegratorMethod=Forward Euler  FilterMethod=Forward Euler  ControllerParametersSource=internal  P=Kp_vq  I=Ki_vq  UseKiTs=off  D=0  UseExternalDerivativeSource=off  N=100  UseFilter=on  TunerSelectOption=Transfer Function Based (PID Tuner App)  InitialConditionSource=internal  InitialConditionForIntegrator=0  InitialConditionForFilter=0  DifferentiatorICPrevScaledInput=0  ExternalReset=none  TrackingMode=off  Kt=1  LimitOutput=on  SatLimitsSource=internal  UpperSaturationLimit=1  LowerSaturationLimit=0  LinearizeAsGain=on  AntiWindupMode=none  Kb=1  LimitIntegrator=off  UpperIntegratorSaturationLimit=inf  LowerIntegratorSaturationLimit=-inf  POutMin=[]  POutMax=[]  IOutMin=[]  IOutMax=[]  DOutMin=[]  DOutMax=[]  NOutMin=[]  NOutMax=[]  SumOutMin=[]  SumOutMax=[]  SaturationOutMin=[]  SaturationOutMax=[]  PParamMin=[]  PParamMax=[]  IParamMin=[]  IParamMax=[]  DParamMin=[]  DParamMax=[]  NParamMin=[]  NParamMax=[]  KbParamMin=[]  KbParamMax=[]  KtParamMin=[]  KtParamMax=[]  KbOutMin=[]  KbOutMax=[]  KtOutMin=[]  KtOutMax=[]  IntegratorOutMin=[]  IntegratorOutMax=[]  FilterOutMin=[]  FilterOutMax=[]  SumI1OutMin=[]  SumI1OutMax=[]  SumI2OutMin=[]  SumI2OutMax=[]  SumI3OutMin=[]  SumI3OutMax=[]  SumI4OutMin=[]  SumI4OutMax=[]  SumDOutMin=[]  SumDOutMax=[]  DifferentiatorOutMin=[]  DifferentiatorOutMax=[]  FilterDiffOutCoefMin=[]  FilterDiffOutCoefMax=[]  ReciprocalOutMin=[]  ReciprocalOutMax=[]  SumDenOutMin=[]  SumDenOutMax=[]  SumNumOutMin=[]  SumNumOutMax=[]  DivideOutMin=[]  DivideOutMax=[]  UdiffTsProdOutMin=[]  UdiffTsProdOutMax=[]  NTsProdOutMin=[]  NTsProdOutMax=[]  UintegralTsProdOutMin=[]  UintegralTsProdOutMax=[]  UngainTsProdOutMin=[]  UngainTsProdOutMax=[]  ClampingZeroOutDataTypeStr=Inherit: Inherit via back propagation  ClampingZeroOutMin=[]  ClampingZeroOutMax=[]  FilterDenConstantOutDataTypeStr=Inherit: Inherit via back propagation  FilterDenConstantOutMin=[]  FilterDenConstantOutMax=[]  PCopyOutDataTypeStr=Inherit: Inherit via back propagation  PCopyOutMin=[]  PCopyOutMax=[]  NCopyOutDataTypeStr=Inherit: Inherit via back propagation  NCopyOutMin=[]  NCopyOutMax=[]  IntegratorContinuousStateAttributes=''  IntegratorStateMustResolveToSignalObject=off  IntegratorRTWStateStorageClass=Auto  FilterContinuousStateAttributes=''  FilterStateMustResolveToSignalObject=off  FilterRTWStateStorageClass=Auto  ParallelPVariant=InternalParameters  IdealPVariant=Disabled  IVariant=InternalParameters  DVariant=Disabled  IntegratorVariant=Discrete  SatVariant=Enabled  AWVariant=Passthrough  PCopyVariant=Disabled  TRVariant=Disabled  FdbkBlocksVariant=Forward  IdealPFdbkVariant=Disabled  SatFdbkVariant=Disabled  DerivativeFilterVariant=Disabled  NVariant=Disabled  NCopyVariant=Disabled_SignalSpec  FilterICVariant=Disabled  IntegratorICVariant=InternalICs  ExternalResetVariant=Disabled  TRSumVariant=Passthrough  SumFdbkVariant=Disabled  SumVariant=Sum_PI  TsampFilterVariant=InternalTs  TsampNgainVariant=Passthrough  TsampIntegralVariant=Disabled_SignalSpec  ExternalSaturationOutDataTypeStr=Inherit: Same as second input  DerivativeSourceVariant=Disabled  PreIntVariant=InternalPreInt
  pu->SI : Gain  Gain=Vrms / sqrt(3) * sqrt(2)
  Vabc_inv : Outport
  ModWave : Outport  Port=2
  tag scope: V_1=global, freq_mea1=global
  wires:
  Vd Discrete PI Controller/1 -> Mux2/1  "Vd inverter"
  Mux2/1 -> Inverse Park Transform/1
  Sum1/1 -> Vd Discrete PI Controller/1
  Park Transform/1 -> Demux/1
  Sum2/1 -> Vq Discrete PI Controller/1
  Demux/2 -> Sum2/1
  Vq Discrete PI Controller/1 -> Mux2/2  "Vq inverter"
  V0/1 -> Mux2/3
  Demux/1 -> Sum1/2
  Demux/3 -> Terminator2/1
  "Sinusoidal Measurement (PLL, Three-Phase)"/3 -> [V_1]
  "Sinusoidal Measurement (PLL, Three-Phase)"/2 -> Inverse Park Transform/2, Park Transform/2
  "Sinusoidal Measurement (PLL, Three-Phase)"/1 -> [freq_mea1]
  Constant/1 -> "PWM Generator (Three-phase, Two-level)"/2
  Inverse Park Transform/1 -> pu->SI/1
  "PWM Generator (Three-phase, Two-level)"/1 -> Unit Delay1/1
  "PWM Generator (Three-phase, Two-level)"/2 -> Unit Delay2/1
  Unit Delay1/1 -> Vabc_inv/1
  pu->SI/1 -> "PWM Generator (Three-phase, Two-level)"/1
  Vabc (pu)/1 -> Power Measurement (Three-Phase)/1, Park Transform/1, "Sinusoidal Measurement (PLL, Three-Phase)"/1
  Iabc (pu)/1 -> Power Measurement (Three-Phase)/2
  Power Measurement (Three-Phase)/1 -> Sum3/2  "Inverter Active Power (pu)"
  Power Measurement (Three-Phase)/2 -> Sum/1  "nverter Reactive Power (pu)"
  P0/1 -> Sum3/1
  Q0/1 -> Sum/2
  Sum/1 -> Kqv/1
  Sum3/1 -> Kpf/1
  Kpf/1 -> Sum5/2
  Kqv/1 -> Sum4/1
  f0/1 -> Sum7/2
  Vref (pu)/1 -> Sum4/2
  Sum7/1 -> Sum5/1
  [freq_mea1] -> Sum7/1
  Sum5/1 -> Sum6/2
  Sum4/1 -> Sum8/2
  [freq_cmd] -> DQ Voltage Reference/1(freq_cmd)
  [V_cmd] -> DQ Voltage Reference/2(V_cmd)
  DQ Voltage Reference/1(Vd_ref) -> Sum1/1
  DQ Voltage Reference/2(Vq_ref) -> Sum2/2
  Unit Delay2/1 -> ModWave/1
  [freq_mea2] -> Transport Delay/1
  [freq_mea1] -> MATLAB Function/1(omega_1)
  Discrete-Time Integrator/1 -> MATLAB Function/6(int_v_in)
  Discrete-Time Integrator1/1 -> MATLAB Function/5(int_w_in)
  [V_1] -> MATLAB Function/3(V_1)
  Constant1/1 -> MATLAB Function/7(Ts)
  MATLAB Function/1(d_omega) -> Gain/1
  MATLAB Function/4(int_v_out) -> Discrete-Time Integrator/1
  MATLAB Function/3(int_w_out) -> Discrete-Time Integrator1/1
  Gain/1 -> Gain1/1
  Sum6/1 -> [freq_cmd]
  Sum8/1 -> [V_cmd]
  MATLAB Function/2(d_V) -> Gain2/1
  Transport Delay/1 -> MATLAB Function/2(omega_2)
  [V_2] -> Transport Delay1/1
  Transport Delay1/1 -> MATLAB Function/4(V_2)
  Gain1/1 -> Scope1/1, Sum6/1  "d_omega1"
  Gain2/1 -> Scope1/2, Sum8/1  "d_V1"

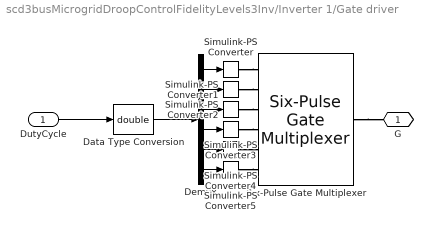
== system scd3busMicrogridDroopControlFidelityLevels3Inv/Inverter 1/Gate driver ==
  DutyCycle : Inport
  Data Type Conversion : DataTypeConversion  OutDataTypeStr=double  SaturateOnIntegerOverflow=off  RndMeth=Floor
  Demux : Demux  Outputs=6
  Simulink-PS Converter{,1..5} (6 alike) : nesl_utility/Simulink-PS Converter  PhysicalDomain=network_engine_domain  SubClassName=ps_input  LeftPortType=input  RightPortType=output  PseudoPeriodic=off  Frequencies=[]  NoiseDistribution=none  NoiseParameters=[]  Unit=1  AffineConversion=off  FilteringAndDerivatives=provide  SimscapeFilterOrder=1  InputFilterTimeConstant=0.001  UdotUserProvided=0
  Six-Pulse Gate Multiplexer : ee_lib/Semiconductors & Converters/Converters/Six-Pulse Gate Multiplexer  port_option=ee.enum.controlport.ps
  G : PMIOPort  Side=Right
  wires:
  Demux/5 -> Simulink-PS Converter4/1
  Demux/3 -> Simulink-PS Converter2/1
  Data Type Conversion/1 -> Demux/1
  Demux/4 -> Simulink-PS Converter3/1
  Demux/6 -> Simulink-PS Converter5/1
  Demux/2 -> Simulink-PS Converter1/1
  Demux/1 -> Simulink-PS Converter/1
  DutyCycle/1 -> Data Type Conversion/1
  connections:
  Simulink-PS Converter4/RConn1 -- Six-Pulse Gate Multiplexer/LConn5
  Simulink-PS Converter2/RConn1 -- Six-Pulse Gate Multiplexer/LConn3
  Simulink-PS Converter/RConn1 -- Six-Pulse Gate Multiplexer/LConn1
  Simulink-PS Converter5/RConn1 -- Six-Pulse Gate Multiplexer/LConn6
  Simulink-PS Converter1/RConn1 -- Six-Pulse Gate Multiplexer/LConn2
  Simulink-PS Converter3/RConn1 -- Six-Pulse Gate Multiplexer/LConn4
  Six-Pulse Gate Multiplexer/RConn1 -- G/RConn1

== system scd3busMicrogridDroopControlFidelityLevels3Inv/Inverter 1/Inverter 1 ==
  Averaged Inverter : Subsystem  VariantControl=AveragedNonSwitch
  IGBT Inverter : Subsystem  VariantControl=PulseSwitch
  + : PMIOPort  Side=Right
  G : PMIOPort  Port=2  Side=Left
  a : PMIOPort  Port=3  Side=Left
  b : PMIOPort  Port=4  Side=Left
  - : PMIOPort  Port=5  Side=Right
  c : PMIOPort  Port=6  Side=Left

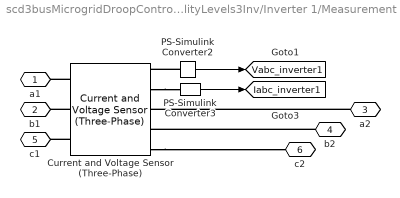
== system scd3busMicrogridDroopControlFidelityLevels3Inv/Inverter 1/Measurement inverter ==
  Current and Voltage Sensor (Three-Phase) : ee_lib/Sensors & Transducers/Current and Voltage Sensor (Three-Phase)  vMeasurementType=2  outputUnit=1  SRated=150000 V*A  VRated=Vrms V  I_specify=off  I_priority=None  I=[ 0 0 0 ] A  I_nominal_specify=off  I_nominal_value=1  I_nominal_unit=A  V_specify=off  V_priority=None  V=[ 0 0 0 ] V  V_nominal_specify=off  V_nominal_value=1  V_nominal_unit=V
      settings: InternalSimscapePortConfiguration="{\"Bottom\":[],\"Left\":[{\"id\":\"a1\",\"label\":\"a1\",\"type\":\"foundation.electrical.electrical\"},{\"id\":\"b1\",\"label\":\"b1\",\"type\":\"foundation.electrical.electrical\"},{\"id\":\"c1\",\"label\":\"c1\",\"type\":\"foundation.electrical.electrical\"}],\"Right\":[{\"id\":\"V_output\",\"label\":\"V\",\"type\":\"output\"},{\"id\":\"I_output\",\"label\":\"I\",\"type\":\"output\"},{\"id\":\"a2\",\"label\":\"a2\",\"type\":\"foundation.electrical.electrical\"},{\"id\":\"b2\",\"label\":\"b2\",\"type\":\"foundation.electrical.electrical\"},{\"id\":\"c2\",\"label\":\"c2\",\"type\":\"foundation.electrical.electrical\"}],\"Top\":[]}"
  PS-Simulink Converter2 : nesl_utility/PS-Simulink Converter  PhysicalDomain=network_engine_domain  SubClassName=ps_output  LeftPortType=input  RightPortType=output  PseudoPeriodic=off  Frequencies=[]  VectorFormat=1-D array  Unit=1  AffineConversion=off
  PS-Simulink Converter3 : nesl_utility/PS-Simulink Converter  PhysicalDomain=network_engine_domain  SubClassName=ps_output  LeftPortType=input  RightPortType=output  PseudoPeriodic=off  Frequencies=[]  VectorFormat=1-D array  Unit=1  AffineConversion=off
  a1 : PMIOPort  Side=Left
  b1 : PMIOPort  Port=2  Side=Left
  a2 : PMIOPort  Port=3  Side=Right
  b2 : PMIOPort  Port=4  Side=Right
  c1 : PMIOPort  Port=5  Side=Left
  c2 : PMIOPort  Port=6  Side=Right
  tag scope: Iabc_inverter1=global, Vabc_inverter1=global
  wires:
  PS-Simulink Converter2/1 -> [Vabc_inverter1]
  PS-Simulink Converter3/1 -> [Iabc_inverter1]
  connections:
  b2/RConn1 -- Current and Voltage Sensor (Three-Phase)/RConn4
  a2/RConn1 -- Current and Voltage Sensor (Three-Phase)/RConn3
  Current and Voltage Sensor (Three-Phase)/RConn5 -- c2/RConn1
  Current and Voltage Sensor (Three-Phase)/LConn2 -- b1/RConn1
  Current and Voltage Sensor (Three-Phase)/LConn3 -- c1/RConn1
  Current and Voltage Sensor (Three-Phase)/LConn1 -- a1/RConn1
  PS-Simulink Converter2/LConn1 -- Current and Voltage Sensor (Three-Phase)/RConn1
  Current and Voltage Sensor (Three-Phase)/RConn2 -- PS-Simulink Converter3/LConn1
